simulink model "simControl"  (R2018b)
settings: Solver=FixedStepAuto  StartTime=0.0  StopTime=30  RelTol=1e-3  EnableMultiTasking=on
settings Model: Creator=mxj6634  LastModifiedBy=axk1188
settings SolverCC: PositivePriorityOrder=on  AutoInsertRateTranBlk=on
settings OptimizationCC: EnhancedBackFolding=on  PassReuseOutputArgsAs=Individual arguments  MaxStackSize=64  OptimizeBlockOrder=speed  DifferentSizesBufferReuse=on  OptimizationCustomize=off
settings DebuggingCC: ParameterTunabilityLossMsg=error
settings HardwareCC: ProdBitPerPointer=32  ProdBitPerSizeT=32  ProdBitPerPtrDiffT=32  ProdLargestAtomicInteger=Long  ProdLargestAtomicFloat=Double  ProdWordSize=32  ProdHWDeviceType=ARM Compatible->ARM Cortex
settings SFSimCC: MATLABDynamicMemAlloc=off
settings RTWCC: SystemTargetFile=ert.tlc  HardwareBoard=Xilinx Zynq-7000 based board  TLCOptions="-aInlineSetEventsForThisBaseRateFcn=TLC_FALSE -aSuppressMultiTaskScheduler=TLC_FALSE  -aRateBasedStepFcn=0"  TemplateMakefile=ert_default_tmf  GenerateReport=on  Toolchain=Linaro AArch32 Linux v6.3.1  IncludeHyperlinkInReport=on  LaunchReport=on  GenerateTraceInfo=on  GenerateTraceReport=on  GenerateTraceReportSl=on  GenerateTraceReportSf=on  GenerateTraceReportEml=on
settings CodeAppCC: ForceParamTrailComments=on  IgnoreCustomStorageClasses=off  OperatorAnnotations=on  SimulinkDataObjDesc=on  SFDataObjDesc=on  InsertBlockDesc=on

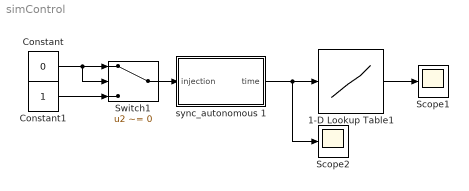
== system simControl ==
  1-D Lookup Table1 : Lookup_n-D  NumberOfTableDimensions=1  BreakpointsForDimension1=[1,2,3,4,5,6,7,8,9]  Table=[0,0,0,0,0,90,0,-90,0]  InternalRulePriority=Speed  RndMeth=Simplest  InputSameDT=on
  Constant : Constant  Value=0
  Constant1 : Constant
  Scope1 : Scope
  Scope2 : Scope
  Switch1 : Switch  Criteria=u2 ~= 0
  sync_autonomous 1 : Subsystem
  wires:
  sync_autonomous 1/1("time ") -> Scope2/1, 1-D Lookup Table1/1
  Switch1/1 -> sync_autonomous 1/1("injection ")
  1-D Lookup Table1/1 -> Scope1/1
  Constant1/1 -> Switch1/3
  Constant/1 -> Switch1/2, Switch1/1

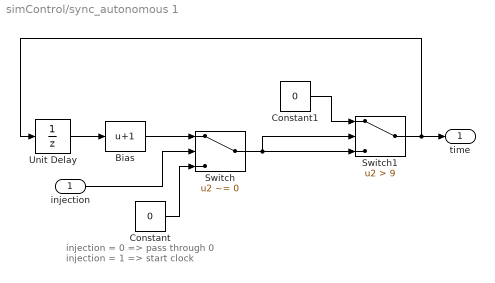
== system simControl/sync_autonomous 1 ==
  note: injection = 0 => pass through 0
      | injection = 1 => start clock
  "injection " : Inport
  Bias : Bias  Bias=1
  Constant : Constant  Value=0  SampleTime=-1
  Constant1 : Constant  Value=0  SampleTime=-1
  Switch : Switch  Criteria=u2 ~= 0
  Switch1 : Switch  Criteria=u2 > Threshold  Threshold=9
  Unit Delay : UnitDelay  SampleTime=-1
  "time " : Outport
  wires:
  Constant/1 -> Switch/3
  Bias/1 -> Switch/1
  "injection "/1 -> Switch/2
  Unit Delay/1 -> Bias/1
  Switch1/1 -> Unit Delay/1, "time "/1
  Switch/1 -> Switch1/3, Switch1/2
  Constant1/1 -> Switch1/1
